simulink model "declination_1"  (R2020b)
settings: Solver=FixedStepAuto  StartTime=1  StopTime=365  FixedStep=1  RelTol=1e-3
libraries: simulink_extras x4
settings Model: Creator=zhiangz  LastModifiedBy=jiang
settings DataIOCC: ReturnWorkspaceOutputs=off
settings DebuggingCC: ArithmeticOperatorsInVariantConditions=warning
settings SFSimCC: SimUseLocalCustomCode=off  CustomCodeUndefinedFunction=UseInterfaceOnly
settings RTWCC: RTWUseLocalCustomCode=off
settings CodeAppCC: StateflowObjectComments=on

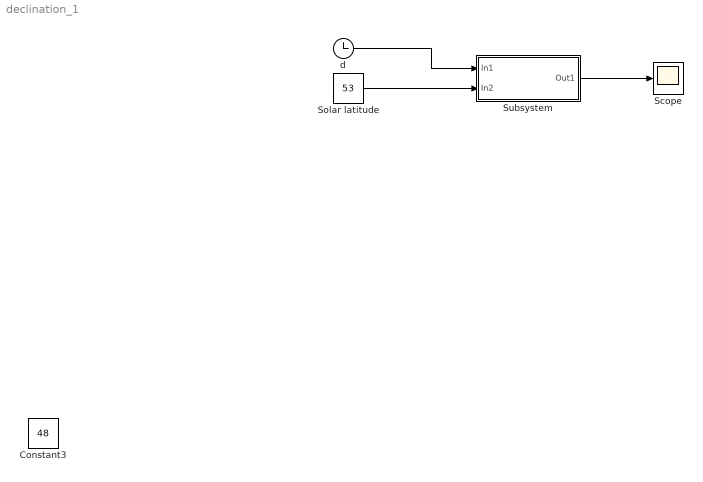
== system declination_1 ==
  Constant3 : Constant  Value=48
  Scope : Scope
  Solar latitude : Constant  Value=53
  Subsystem : Subsystem
  d : Clock
      settings: Decimation=365
  wires:
  ? -> ?
  d/1 -> Subsystem/1(In1)
  Solar latitude/1 -> Subsystem/2(In2)
  Subsystem/1(Out1) -> Scope/1

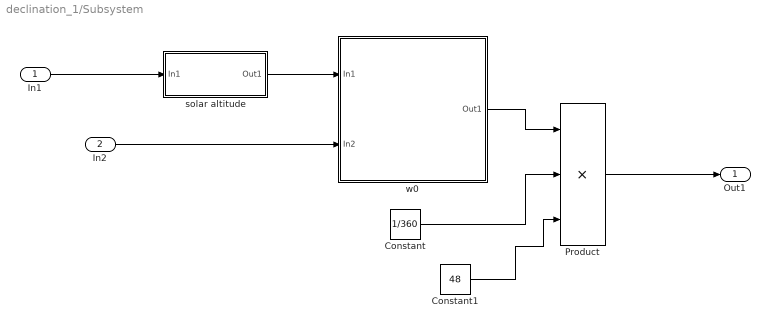
== system declination_1/Subsystem ==
  In1 : Inport
  In2 : Inport  Port=2
  Constant : Constant  Value=1/360
  Constant1 : Constant  Value=48
  Product : Product  Inputs=3
  solar altitude : Subsystem
  w0 : Subsystem
  Out1 : Outport
  wires:
  w0/1(Out1) -> Product/1
  solar altitude/1(Out1) -> w0/1(In1)
  Constant/1 -> Product/2
  Constant1/1 -> Product/3
  In1/1 -> solar altitude/1(In1)
  In2/1 -> w0/2(In2)
  Product/1 -> Out1/1

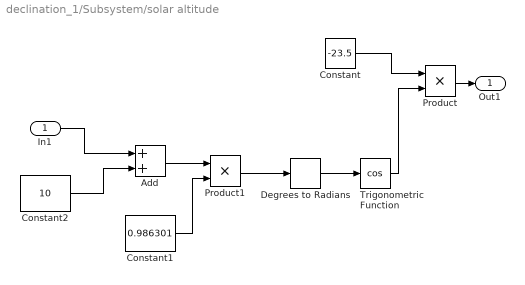
== system declination_1/Subsystem/solar altitude ==
  In1 : Inport
  Add : Sum
  Constant : Constant  Value=-23.5
  Constant1 : Constant  Value=0.986301
  Constant2 : Constant  Value=10
  Degrees to Radians : simulink_extras/Transformations/Degrees to Radians
  Product : Product
  Product1 : Product
  Trigonometric Function : Trigonometry  Operator=cos
  Out1 : Outport
  wires:
  Constant1/1 -> Product1/2
  Add/1 -> Product1/1
  Degrees to Radians/1 -> Trigonometric Function/1
  Trigonometric Function/1 -> Product/2
  Product1/1 -> Degrees to Radians/1
  Constant2/1 -> Add/2
  Constant/1 -> Product/1
  In1/1 -> Add/1
  Product/1 -> Out1/1

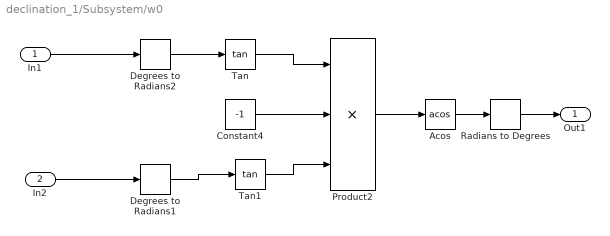
== system declination_1/Subsystem/w0 ==
  In1 : Inport
  In2 : Inport  Port=2
  Acos : Trigonometry  Operator=acos
  Constant4 : Constant  Value=-1
  Degrees to Radians1 : simulink_extras/Transformations/Degrees to Radians
  Degrees to Radians2 : simulink_extras/Transformations/Degrees to Radians
  Product2 : Product  Inputs=3
  Radians to Degrees : simulink_extras/Transformations/Radians to Degrees
  Tan : Trigonometry  Operator=tan
  Tan1 : Trigonometry  Operator=tan
  Out1 : Outport
  wires:
  Tan/1 -> Product2/1
  In2/1 -> Degrees to Radians1/1
  Tan1/1 -> Product2/3
  Degrees to Radians1/1 -> Tan1/1
  Degrees to Radians2/1 -> Tan/1
  In1/1 -> Degrees to Radians2/1
  Constant4/1 -> Product2/2
  Product2/1 -> Acos/1
  Acos/1 -> Radians to Degrees/1
  Radians to Degrees/1 -> Out1/1
